simulink model "me13"  (R2023a)
settings: Solver=VariableStepAuto  StartTime=0.0  StopTime=10.0  RelTol=1e-3
values from neighbouring files (symbols this model uses):
  alfa = (1-sin(fi_rad)) / (1+sin(fi_rad))    [proracun.m]
  T = 1 / (sqrt(alfa) * w_c)    [proracun.m]
  Ts = 0    [proracun.m]
undefined symbols (not defined in the file or in its folder): Serial_Port, Standard_Devices
libraries: simulink x3, sldrtlib x2
settings Model: Creator=pavij  LastModifiedBy=pavij

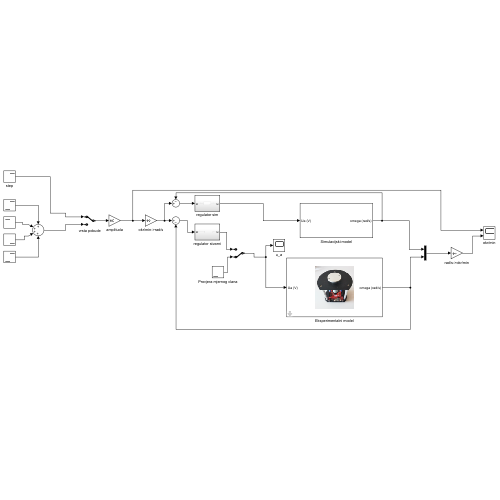
[thumbnail: Simulink's stored preview of the top-level diagram]
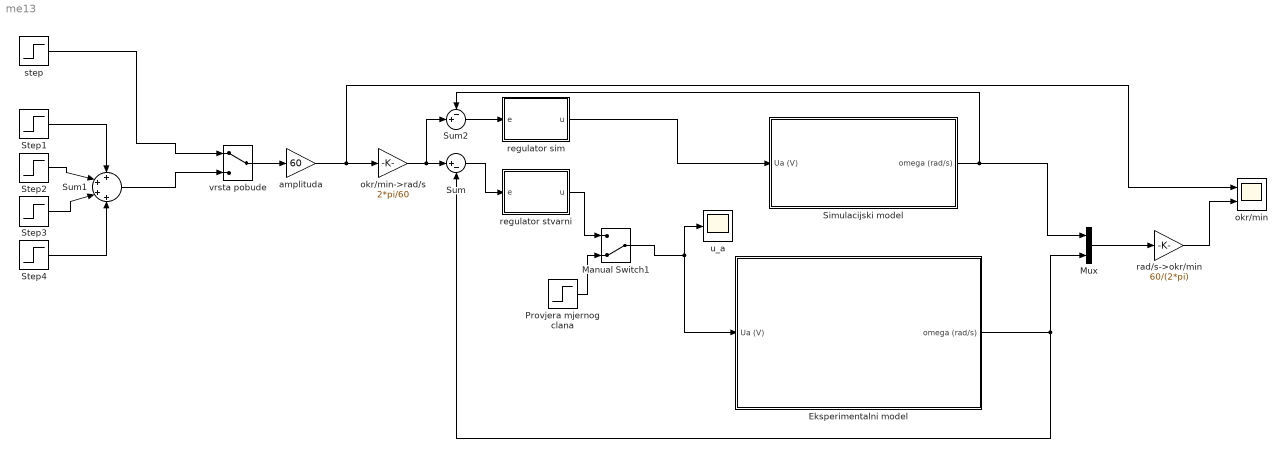
== system me13 ==
  Eksperimentalni model : Subsystem  mask{R6=383, motorRes=2849.3, Ts=Ts}
      mask init:
      | % currentBlock = gcb;
      | % ud = get_param(gcb,'UserData');
      | % %% LIST ALL THE COM PORTS AND TRY TO COMMUNICATE!
      | % if ud.i == 0
      | %     %% Closing all the ports:
      | %     Port = '';
      | %     FullPort = '';
      | %     if ~isempty(instrfind)
      | %         fclose(instrfind);
      | %         delete(instrfind);
      | %     end
      | %     %% Find all the COM ports in a computer
      | %     s1 = instrhwinfo('serial');
      | %     for i = 1:length(s1.AvailableSerialPorts)
      | %         s = serial(s1.AvailableSerialPorts{i});
      | %         set(s, 'BaudRate', 115200);
      | %         pause(0.01)
      | %         j = 0;
      | %         while (contains(s.status,'closed','IgnoreCase',true) && j < 2)
      | %             %% Try to open the port
      | %             j = j+1;
      | %             fopen(s);
      | %             pause(0.01)
      | %         end
      | %         if contains(s.status,'open','IgnoreCase',true && s.BytesAvailable > 14)
      | %             for j = 1:2
      | %                 %if s.BytesAvailable > 0
      | %                 pause(1)
      | %                 readData = fscanf(s);
      | %                 %end
      | %                 pause(0.01)
      | %                 
      | %                 if contains(readData,'BARBELL','IgnoreCase',true)
      | %                     disp(['Barbell Lab control board is on port: ', s1.AvailableSerialPorts{i}]);
      | %                     Port = s1.AvailableSerialPorts{i};
      | %                     while (s.BytesAvailable >0)
      | %                         readData = fscanf(s);
      | %                     end
      | %                     readData = '';
      | %                     
      | %                     %%
      | %                     fprintf(s, "%c%c%c%c", char(typecast(int16([32767 2]),'uint8')));
      | %                     while(s.BytesAvailable > 10)
      | %                         b = fread(s,5,'int16');
      | %                     end
      | %                     fprintf(s, "%c%c%c%c", char(typecast(int16([0 0]),'uint8')));
      | %                     while(s.BytesAvailable > 10)
      | %                         b = fread(s,5,'int16');
      | %                     end
      | %                     break;
      | %                 end
      | %             end
      | %             
      | %             
      | %             fclose(s);
      | %             
      | %         end
      | %         if (~isempty(Port))
      | %             break;
      | %         end
      | %     end
      | %     if (isempty(Port))
      | %      %   msgbox('Barbell lab board not found, make sure it is connected, FTDI driver is installed and try again')
      | %     else
      | %         %% Set Packet Input and Packet Output parameters
      | %         po = strcat(currentBlock,'/Packet Output1');
      | %         pinput = strcat(currentBlock,'/Packet Input1');
      | %         %%
      | %         set_param(po, 'LinkStatus','inactive');
      | %         set_param(pinput, 'LinkStatus','inactive');
      | %         %%
      | %         p = Simulink.Mask.get(po);
      | %         a = p.Parameters(6);
      | %         FullPort = Port;
      | %         Port = replace(Port,'COM','');
      | %         if length(Port)==0
      | %             Port = a.Value
      | %         end
      | %         %%
      | %         
      | %         a.set('Value',Port);
      | %         %%
      | %         %%
      | %         %%
      | %         p1 = Simulink.Mask.get(pinput);
      | %         a1 = p1.Parameters(6);
      | %         a1.set('Value',Port);
      | %         
      | %         
      | %         %% Latency configuration
      | %         %% Check if PORT FOUND
      | %         if (isempty(Port))
      | %             disp('Barbell lab board not found')
      | %         else
      | %             
      | %             %% Check if Windows FTDI driver is used!
      | %             [ok,txt] = system('reg query HKEY_LOCAL_MACHINE\SYSTEM\CurrentControlSet\Enum\FTDIBUS');
      | %             newStr = splitlines(txt);
      | %             %%
      | %             brojac = 0;
      | %             found = 0;
      | %             for i = 1:size(newStr,1)
      | %                 if ~isempty(newStr{i})
      | %                     %%
      | %                     brojac = brojac +1;
      | %                     tmp = [newStr{i} '\0000\Device Parameters'];
      | %                     tmp1{brojac} = strrep(tmp,'HKEY_LOCAL_MACHINE\','');
      | %                     portName{brojac} = winqueryreg('HKEY_LOCAL_MACHINE',tmp1{brojac},'PortName');
      | %                     value{brojac} = winqueryreg('HKEY_LOCAL_MACHINE',tmp1{brojac},'LatencyTimer');
      | %                     tmpvalue = value{brojac};
      | %                     if (strcmp(portName{brojac}, FullPort))
      | %                         found = 1;
      | %                         break;
      | %                     end
      | %                 end
      | %             end
      | %             %%
      | %             if found == 0
      | %                 msgbox(['FTDI driver not found, please adjust the latency of ',FullPort,' manually'])
      | %                 disp('FTDI driver not found!')
      | %                 system('mmc devmgmt.msc')
      | %             else
      | %                 %% Widnows FTDI driver is used
      | %                 if tmpvalue > 2
      | %                     %% If Latency timer is greater than 2
      | %                     str = [ud.bat,...
      | %                         'reg add "', tmp, '" /v LatencyTimer /t REG_DWORD /d 00000001 /f    ',char(10)];
      | %                     %%
      | %                     disp('Attempting to change the Latency timer value')
      | %                     try
      | %                         fileID = fopen('bblt.bat','w');
      | %                         fprintf(fileID, '%s', str);
      | %                         fclose(fileID);
      | %                     catch
      | %                         msgbox(['Insufficient permissions, please adjust the latency of ',FullPort,' manually'])
      | %                         system('mmc devmgmt.msc')
      | %                         a = 0;
      | %                     end
      | %                     %%
      | %                     system('bblt.bat')
      | %                     
      | %                     %             if exist('bblt.bat', 'file')==2
      | %                     %                 delete('bblt.bat');
      | %                     %             end
      | %                 end
      | %             end
      | %         end
      | %     end
      | % end
      | % ud.i = ud.i + 1;
      | % if ud.i == 2
      | %     ud.i = 0;
      | % end
      | % set_param(gcb, 'UserData',ud)
      mask Display:
      | ud = get_param(gcb,'UserData');
      | image(ud.x);
  Manual Switch1 : ManualSwitch  CurrentSetting=0
  Mux : Mux  Inputs=2
  Provjera mjernog clana : Step  Time=2  After=3  SampleTime=0
  Simulacijski model : Subsystem
      mask init: same as me13/Eksperimentalni model
  Step1 : Step  Time=2  SampleTime=0
  Step2 : Step  Time=4  After=-1  SampleTime=0
  Step3 : Step  Time=6  After=-1  SampleTime=0
  Step4 : Step  Time=8  SampleTime=0
  Sum : Sum  Inputs=|+-
  Sum1 : Sum  Inputs=++++
  Sum2 : Sum  Inputs=-+|
  amplituda : Gain  Gain=60
  okr/min : Scope  NumInputPorts=2
  okr/min->rad/s : Gain  Gain=2*pi/60
  rad/s->okr/min : Gain  Gain=60/(2*pi)
  regulator sim : Subsystem
  regulator stvarni : Subsystem
  step : Step  Time=2  SampleTime=0
  u_a : Scope
  vrsta pobude : ManualSwitch
  wires:
  Step2/1 -> Sum1/2
  Manual Switch1/1 -> u_a/1, Eksperimentalni model/1(Ua (V))
  regulator sim/1(u) -> Simulacijski model/1(Ua (V))
  Eksperimentalni model/1(omega (rad/s)) -> Sum/2, Mux/2
  amplituda/1 -> okr/min/1, okr/min->rad/s/1
  rad/s->okr/min/1 -> okr/min/2
  vrsta pobude/1 -> amplituda/1
  regulator stvarni/1(u) -> Manual Switch1/1
  Sum2/1 -> regulator sim/1(e)
  Simulacijski model/1(omega (rad/s)) -> Mux/1, Sum2/1
  Sum/1 -> regulator stvarni/1(e)
  Provjera mjernog clana/1 -> Manual Switch1/2
  Mux/1 -> rad/s->okr/min/1
  Step3/1 -> Sum1/3
  Step1/1 -> Sum1/1
  step/1 -> vrsta pobude/1
  okr/min->rad/s/1 -> Sum/1, Sum2/2
  Step4/1 -> Sum1/4
  Sum1/1 -> vrsta pobude/2

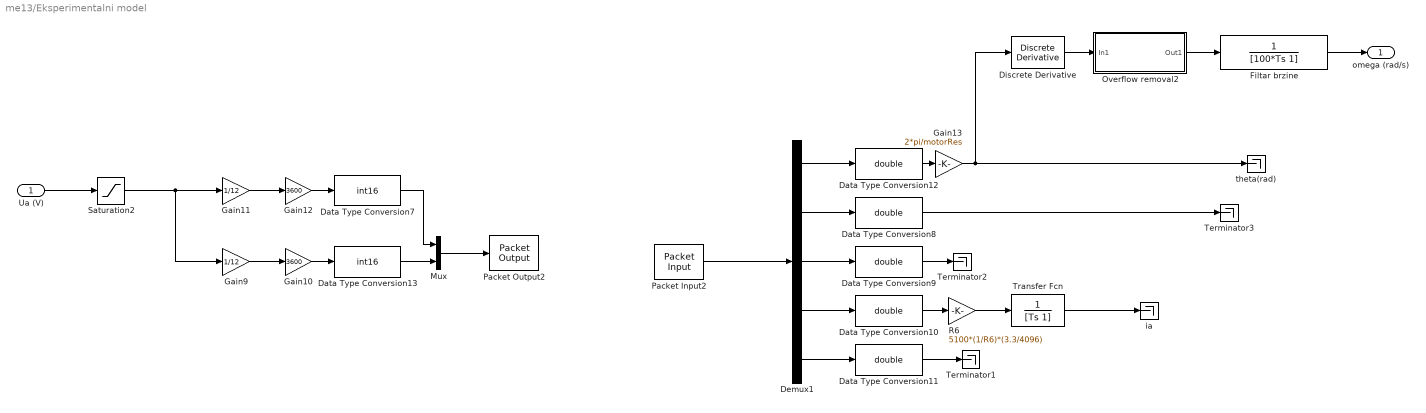
== system me13/Eksperimentalni model ==
  Ua (V) : Inport
  Data Type Conversion{8..12} (5 alike) : DataTypeConversion  OutDataTypeStr=double  SaturateOnIntegerOverflow=off  RndMeth=Floor
  Data Type Conversion13 : DataTypeConversion  OutDataTypeStr=int16  SaturateOnIntegerOverflow=off  RndMeth=Floor
  Data Type Conversion7 : DataTypeConversion  OutDataTypeStr=int16  SaturateOnIntegerOverflow=off  RndMeth=Floor
  Demux1 : Demux  Outputs=5
  Discrete Derivative : simulink/Discrete/Discrete Derivative  gainval=1.0  ICPrevScaledInput=0.0  OutMin=[]  OutMax=[]  OutDataType=fixdt(1, 16)  OutScaling=2^-10  DoSatur=off
  Filtar brzine : TransferFcn  Denominator=[100*Ts 1]
  Gain10 : Gain  Gain=3600
  Gain11 : Gain  Gain=1/12
  Gain12 : Gain  Gain=3600
  Gain13 : Gain  Gain=2*pi/motorRes  OutDataTypeStr=double
  Gain9 : Gain  Gain=1/12
  Mux : Mux  Inputs=2
  Overflow removal2 : Subsystem
  Packet Input2 : sldrtlib/Packet Input  SampleTime=Ts  MaxMissedTicks=10  ShowMissedTicks=off  YieldWhenWaiting=off  DrvName=Standard_Devices/Serial_Port  DrvAddress=3  DrvOptions=[115200 8 0 0 0 0 0 0]  PacketSize=5*2  DataTypes='5*int16'  ShowReady=off  ShowError=off  PacketID=1  ByteOrder=1  ShowTimestamp=off
      settings: AttributesFormatString=Serial Port [3]
  Packet Output2 : sldrtlib/Packet Output  SampleTime=Ts  MaxMissedTicks=10  ShowMissedTicks=off  YieldWhenWaiting=off  DrvName=Standard_Devices/Serial_Port  DrvAddress=3  DrvOptions=[115200 8 0 0 0 0 0 0]  PacketSize=4  DataTypes='2*int16'  ShowReady=off  ShowError=off  PacketID=1  ByteOrder=1  InitialValue=[32767 2]  FinalValue=[0 0]
      settings: AttributesFormatString=Serial Port [3]
  R6 : Gain  Gain=5100*(1/R6)*(3.3/4096)
  Saturation2 : Saturate  UpperLimit=12  LowerLimit=-12
  Terminator1 : Terminator
  Terminator2 : Terminator
  Terminator3 : Terminator
  Transfer Fcn : TransferFcn  Denominator=[Ts 1]
  ia : Terminator
  theta(rad) : Terminator
  omega (rad/s) : Outport  VectorParamsAs1DForOutWhenUnconnected=off
  wires:
  Ua (V)/1 -> Saturation2/1
  Gain12/1 -> Data Type Conversion7/1
  Gain11/1 -> Gain12/1
  Gain10/1 -> Data Type Conversion13/1
  Gain9/1 -> Gain10/1
  Demux1/1 -> Data Type Conversion12/1
  Demux1/2 -> Data Type Conversion8/1
  Demux1/3 -> Data Type Conversion9/1
  Demux1/4 -> Data Type Conversion10/1
  Demux1/5 -> Data Type Conversion11/1
  Saturation2/1 -> Gain9/1, Gain11/1
  Data Type Conversion7/1 -> Mux/1
  Data Type Conversion13/1 -> Mux/2
  Data Type Conversion8/1 -> Terminator3/1
  Data Type Conversion12/1 -> Gain13/1
  Gain13/1 -> theta(rad)/1, Discrete Derivative/1
  Discrete Derivative/1 -> Overflow removal2/1(In1)
  Filtar brzine/1 -> omega (rad/s)/1
  Mux/1 -> Packet Output2/1
  Data Type Conversion11/1 -> Terminator1/1
  Data Type Conversion10/1 -> R6/1
  Data Type Conversion9/1 -> Terminator2/1
  R6/1 -> Transfer Fcn/1
  Overflow removal2/1(Out1) -> Filtar brzine/1
  Packet Input2/1 -> Demux1/1
  Transfer Fcn/1 -> ia/1

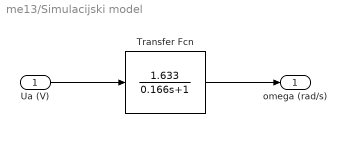
== system me13/Simulacijski model ==
  Ua (V) : Inport
  Transfer Fcn : TransferFcn  Numerator=[1.633]  Denominator=[0.166 1]
  omega (rad/s) : Outport  VectorParamsAs1DForOutWhenUnconnected=off
  wires:
  Ua (V)/1 -> Transfer Fcn/1
  Transfer Fcn/1 -> omega (rad/s)/1

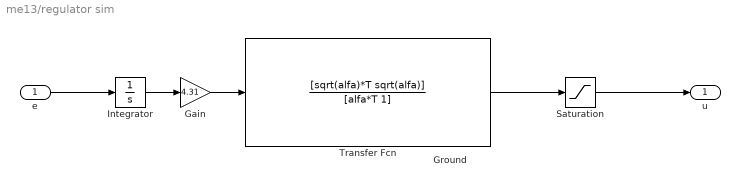
== system me13/regulator sim ==
  e : Inport
  Gain : Gain  Gain=4.31
  Ground : Ground
  Integrator : Integrator
  Saturation : Saturate  UpperLimit=6  LowerLimit=-6
  Transfer Fcn : TransferFcn  Numerator=[sqrt(alfa)*T sqrt(alfa)]  Denominator=[alfa*T 1]
  u : Outport
  wires:
  Saturation/1 -> u/1
  Gain/1 -> Transfer Fcn/1
  Integrator/1 -> Gain/1
  Transfer Fcn/1 -> Saturation/1
  e/1 -> Integrator/1

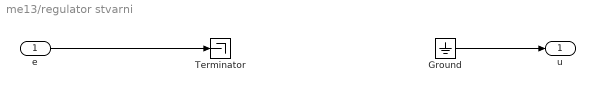
== system me13/regulator stvarni ==
  e : Inport
  Ground : Ground
  Terminator : Terminator
  u : Outport
  wires:
  Ground/1 -> u/1
  e/1 -> Terminator/1

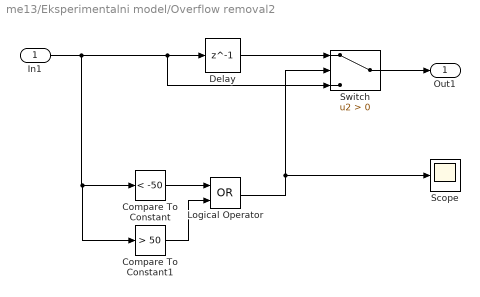
== system me13/Eksperimentalni model/Overflow removal2 ==
  In1 : Inport
  Compare To Constant : simulink/Logic and Bit Operations/Compare To Constant  relop=<  const=-50  OutDataTypeStr=boolean
  Compare To Constant1 : simulink/Logic and Bit Operations/Compare To Constant  relop=>  const=50  OutDataTypeStr=boolean
  Delay : Delay  DelayLength=1  InitialCondition=0  UseCircularBuffer=on
  Logical Operator : Logic  Operator=OR  AllPortsSameDT=off  OutDataTypeStr=boolean
  Scope : Scope
  Switch : Switch  Criteria=u2 > Threshold  SaturateOnIntegerOverflow=off  InputSameDT=off
  Out1 : Outport  VectorParamsAs1DForOutWhenUnconnected=off
  wires:
  In1/1 -> Switch/3, Delay/1, Compare To Constant1/1, Compare To Constant/1
  Compare To Constant/1 -> Logical Operator/1
  Compare To Constant1/1 -> Logical Operator/2
  Delay/1 -> Switch/1
  Switch/1 -> Out1/1
  Logical Operator/1 -> Scope/1, Switch/2
